simulink model "P3_Modelo_4_7_MotorReal"  (R2025b)
settings: Solver=VariableStepAuto  StartTime=0.0  StopTime=10.0  RelTol=1e-3
undefined symbols (not defined in the file): K, k_e, p
libraries: simulink x1
settings Model: Creator=Pc24
settings DebuggingCC: UnconnectedInputMsg=warning  UnconnectedOutputMsg=warning  UnconnectedLineMsg=warning
settings ModelReferenceCC: EnableRefExpFcnMdlSchedulingChecks=on
settings RTWCC: GPUComputeCapability=3.5  DLArmComputeVersion=19.05

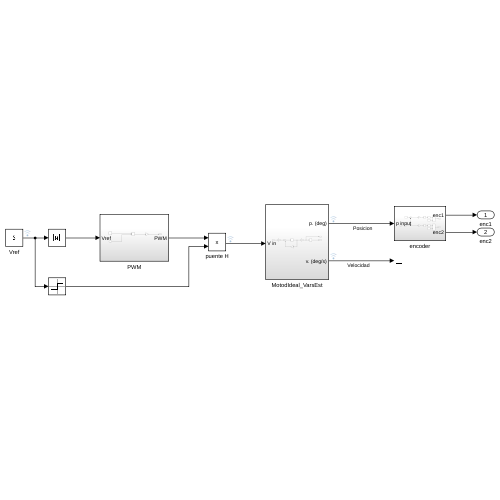
[thumbnail: Simulink's stored preview of the top-level diagram]
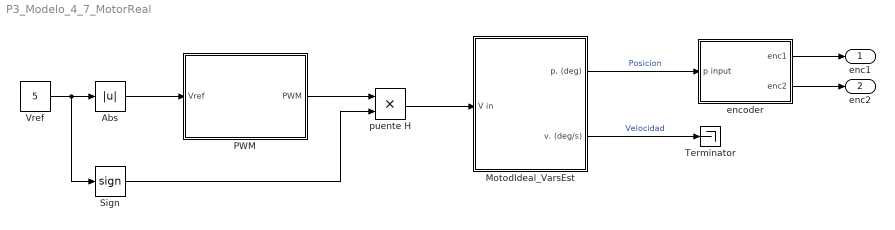
== system P3_Modelo_4_7_MotorReal ==
  Abs : Abs  SaturateOnIntegerOverflow=off
  MotodIdeal_VarsEst : Subsystem
  PWM : Subsystem
  Sign : Signum
  Terminator : Terminator
  Vref : Constant  Value=5
  encoder : Subsystem
  puente H : Product
  enc1 : Outport
  enc2 : Outport  Port=2
  wires:
  MotodIdeal_VarsEst/1(p. (deg)) -> encoder/1(p input)  "Posicion"
  encoder/1(enc1) -> enc1/1
  encoder/2(enc2) -> enc2/1
  Vref/1 -> Sign/1, Abs/1
  Sign/1 -> puente H/2
  puente H/1 -> MotodIdeal_VarsEst/1(V in)
  MotodIdeal_VarsEst/2(v. (deg/s)) -> Terminator/1  "Velocidad"
  PWM/1(PWM) -> puente H/1
  Abs/1 -> PWM/1(Vref)

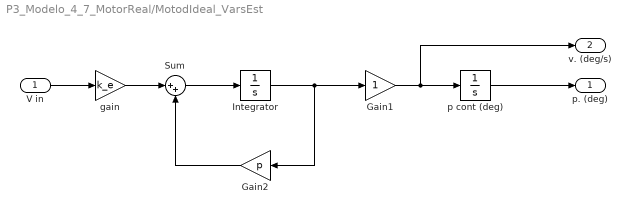
== system P3_Modelo_4_7_MotorReal/MotodIdeal_VarsEst ==
  V in : Inport
  Gain1 : Gain
  Gain2 : Gain  Gain=p
  Integrator : Integrator
  Sum : Sum  Inputs=|++
  gain : Gain  Gain=k_e
  p cont (deg) : Integrator
  p. (deg) : Outport
  v. (deg/s) : Outport  Port=2
  wires:
  gain/1 -> Sum/1
  Gain1/1 -> v. (deg/s)/1, p cont (deg)/1
  Integrator/1 -> Gain2/1, Gain1/1
  p cont (deg)/1 -> p. (deg)/1
  Gain2/1 -> Sum/2
  Sum/1 -> Integrator/1
  V in/1 -> gain/1

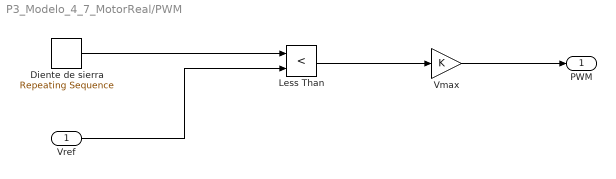
== system P3_Modelo_4_7_MotorReal/PWM ==
  Vref : Inport
  Diente de sierra : simulink/Sources/Repeating Sequence  rep_seq_t=[0 2]  rep_seq_y=[0 2]
  Less Than : RelationalOperator  Operator=<  OutDataTypeStr=boolean  RndMeth=Simplest  InputSameDT=off
  Vmax : Gain  Gain=K
  PWM : Outport
  wires:
  Diente de sierra/1 -> Less Than/1
  Vmax/1 -> PWM/1
  Vref/1 -> Less Than/2
  Less Than/1 -> Vmax/1

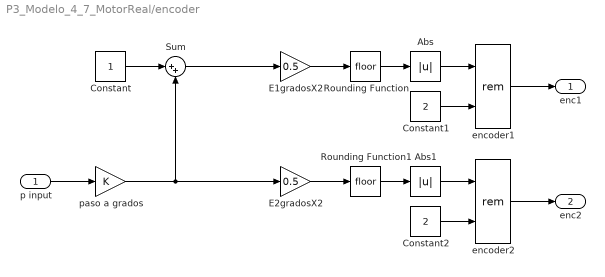
== system P3_Modelo_4_7_MotorReal/encoder ==
  p input : Inport
  Abs : Abs  SaturateOnIntegerOverflow=off
  Abs1 : Abs  SaturateOnIntegerOverflow=off
  Constant : Constant
  Constant1 : Constant  Value=2
  Constant2 : Constant  Value=2
  E1gradosX2 : Gain  Gain=0.5
  E2gradosX2 : Gain  Gain=0.5
  Rounding Function : Rounding
  Rounding Function1 : Rounding
  Sum : Sum  Inputs=|++
  encoder1 : Math  Operator=rem
  encoder2 : Math  Operator=rem
  paso a grados : Gain  Gain=K
  enc1 : Outport
  enc2 : Outport  Port=2
  wires:
  Constant2/1 -> encoder2/2
  Abs1/1 -> encoder2/1
  paso a grados/1 -> E2gradosX2/1, Sum/2
  Abs/1 -> encoder1/1
  E1gradosX2/1 -> Rounding Function/1
  encoder1/1 -> enc1/1
  Rounding Function/1 -> Abs/1
  Constant/1 -> Sum/1
  encoder2/1 -> enc2/1
  p input/1 -> paso a grados/1
  E2gradosX2/1 -> Rounding Function1/1
  Sum/1 -> E1gradosX2/1
  Constant1/1 -> encoder1/2
  Rounding Function1/1 -> Abs1/1
